simulink model "free_motion_model"  (R2021b)
settings: Solver=VariableStepAuto  StartTime=0.0  StopTime=10.0  RelTol=1e-3
undefined symbols (not defined in the file): a_0, a_1
settings Model: Creator=den  LastModifiedBy=den

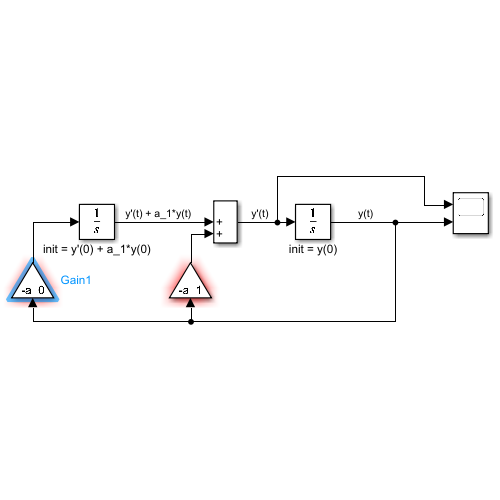
[thumbnail: Simulink's stored preview of the top-level diagram]
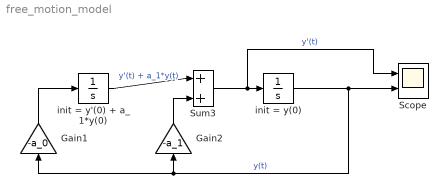
== system free_motion_model ==
  Gain1 : Gain  Gain=-a_0
  Gain2 : Gain  Gain=-a_1
  Scope : Scope  NumInputPorts=2
  Sum3 : Sum  Inputs=|++
  init = y'(0) + a_1*y(0) : Integrator  InitialCondition=6
  init = y(0) : Integrator  InitialCondition=1
  wires:
  init = y(0)/1 -> Gain1/1, Gain2/1, Scope/2  "y(t)"
  Sum3/1 -> Scope/1, init = y(0)/1  "y'(t)"
  Gain1/1 -> init = y'(0) + a_1*y(0)/1
  init = y'(0) + a_1*y(0)/1 -> Sum3/1  "y'(t) + a_1*y(t)"
  Gain2/1 -> Sum3/2
